simulink model "ID_3d_pend"  (R2023a)
settings: Solver=VariableStepAuto  StartTime=0.0  StopTime=1  RelTol=1e-9  AbsTol=1e-9  EnableMultiTasking=on
values from neighbouring files (symbols this model uses):
  a_el = [r_ej,h_ej,r_ej]    [data.m]
  akt = [0.5,0.5]*1    [inverse_dynamics.m]    (also in odvozeni_svaly.m = sym('akt',[1 3]))
  ax = r_ej    (= 0.088)    [data.m]
  ay = h_ej    (= 0.15)    [data.m]
  az = r_ej    (= 0.088)    [data.m]
  ccom = [-0.0110972, 0.00637508, 0.0541825]    [data.m]    (also in fo_python_to_matlab.m = [ccomx, ccomy, ccomz]; mm_python_to_matlab.m = [ccomx, ccomy, ccomz])
  cI = [5.75482e-05, 6.05521e-05, 1.05345e-05,-1.27405e-05, 1.65861e-05, 4.50136e-06]    [data.m]    (also in mm_python_to_matlab.m = [cixx, ciyy, cizz, cixy, ciyz, cizx])
  cont1 = [-0.083529 -0.01368 -0.098954]-scom    [data.m]
  cont2 = [-0.105456 -0.125076 -0.075251]-scom    [data.m]
  cont_params = [k_contact, eps]    [data.m]
  force = [556.8,1098.4]    [inverse_dynamics.m]    (also in odvozeni_svaly.m = (((length / l0m)^3) * exp(8 * length / l0m - 12.9) + (exp(-()
  h_ej = 0.15    [data.m]
  hcom = [0.000389382, -0.116338, -0.00231072]    [data.m]    (also in fo_python_to_matlab.m = [hcomx, hcomy, hcomz]; mm_python_to_matlab.m = [hcomx, hcomy, hcomz])
  hI = [0.00326632, 4.34807e-05, 0.00325004,-0.000136456, -1.30958e-06, -1.14964e-05]    [data.m]    (also in mm_python_to_matlab.m = [hixx, hiyy, hizz, hixy, hiyz, hizx])
  initialConditions = zeros(1,18)    [inverse_dynamics.m]
  k_contact = 10000    [data.m]
  l0m = [0.152404782147249,0.0902153118932702]    [inverse_dynamics.m]
  m = [0.0370005,0.12759,0.26363]    [data.m]    (also in fo_python_to_matlab.m = [c_m,s_m,h_m]; mm_python_to_matlab.m = [c_m,s_m,h_m])
  m_el = [x_ej,y_ej,z_ej]    [data.m]
  mx = x_ej    (= -0.03)    [data.m]
  my = y_ej    (= -0.1)    [data.m]
  mz = z_ej    (= 0.05)    [data.m]
  p = [c,k,g]    [data.m]    (also in fo_python_to_matlab.m)
  r_ej = 0.088    [data.m]
  scom = [-0.0512948, -0.0367122, -0.0430756]    [data.m]    (also in fo_python_to_matlab.m = [scomx, scomy, scomz]; mm_python_to_matlab.m = [scomx, scomy, scomz])
  sI = [0.00020065, 0.000202939, 0.000227237,-4.55661e-05, -7.53511e-05, -7.42694e-05]    [data.m]    (also in mm_python_to_matlab.m = [sixx, siyy, sizz, sixy, siyz, sizx])
  T_c = [-0.01433 0.02007 0.135535]    [data.m]    (also in fo_python_to_matlab.m = [T_cx,T_cy,T_cz]; mm_python_to_matlab.m = [T_cx,T_cy,T_cz]; odvozeni_svaly.m)
  T_d = 1e-20    [data.m]
  T_s = [-0.00955 -0.034 0.009]    [data.m]    (also in fo_python_to_matlab.m = [T_sx,T_sy,T_sz]; mm_python_to_matlab.m = [T_sx,T_sy,T_sz]; odvozeni_svaly.m)
  T_t = [0.006325 0.00693 0.025465]    [data.m]    (also in odvozeni_svaly.m)
  x_ej = -0.03    [data.m]
  y_ej = -0.1    [data.m]
  z_ej = 0.05    [data.m]
undefined symbols (not defined in the file or in its folder): phi_0, r_0, r_10, r_20, X, Y, Z
libraries: sm_lib x68, nesl_utility x43
(part 3 of 3)

== matlab function ID_3d_pend/MATLAB Function1 ==
  data: t input; q output
function q  = fcn(t)
% 
q = 0.2*cos(3*t)-0.1;
% dq = -0.5*sin(1*t);
% ddq = -0.5*cos(1*t);
% q = 0;
% dq = 0;
% ddq = 0;

== matlab function ID_3d_pend/scapulohumeral_rhythm/1_point_contact/r = fcn(h) ==
  data: h input; r output; h_ej parameter; r_ej parameter
function r = fcn(h,h_ej,r_ej)

r = sqrt((r_ej^2)*(1-h^2/h_ej^2));

== matlab function ID_3d_pend/scapulohumeral_rhythm/2_points_contact/ellipsoidal_joint_1/r = fcn(h) ==
  data: h input; r output; h_ej parameter; r_ej parameter
function r = fcn(h,h_ej,r_ej)

r = sqrt((r_ej^2)*(1-h^2/h_ej^2));

== matlab function ID_3d_pend/scapulohumeral_rhythm/2_points_contact/ellipsoidal_joint_2/r = fcn(h) ==
  data: h input; r output; h_ej parameter; r_ej parameter
function r = fcn(h,h_ej,r_ej)

r = sqrt((r_ej^2)*(1-h^2/h_ej^2));

== matlab function ID_3d_pend/MATLAB Function2 ==
  data: x1 input; xx output; x2 input; x3 input; x4 input; x5 input; x6 input; T_t parameter; T_c parameter; scom parameter; cont1 parameter; cont2 parameter; k_contact parameter; eps parameter; ax parameter; ay parameter; az parameter; mx parameter; my parameter; mz parameter
function xx = fcn(x1,x2,x3,x4,x5,x6,T_t, T_c, scom,cont1,cont2,k_contact, eps, ax, ay, az, mx, my, mz)
T_tx=T_t(1);
T_ty=T_t(2);
T_tz=T_t(3);
T_cx = T_c(1);
T_cy = T_c(2);
T_cz = T_c(3);
scomx = scom(1);
scomy = scom(2);
scomz = scom(3);
x_cont1 = cont1(1);
y_cont1 = cont1(2);
z_cont1 = cont1(3);
x_cont2 = cont2(1);
y_cont2 = cont2(2);
z_cont2 = cont2(3);

xx = -k_contact.*(ax.^2 + ay.^2 + az.^2).*(-0.5*sqrt(eps.^2 + (-1 + (T_cx.*(sin(x1).*sin(x3) - sin(x2).*cos(x1).*cos(x3)) + T_cy.*(sin(x1).*cos(x3) + sin(x2).*sin(x3).*cos(x1)) + T_cz.*cos(x1).*cos(x2) + T_tz - mz + scomx.*((sin(x1).*sin(x3) - sin(x2).*cos(x1).*cos(x3)).*cos(x5).*cos(x6) + (sin(x1).*cos(x3) + sin(x2).*sin(x3).*cos(x1)).*(sin(x4).*sin(x5).*cos(x6) + sin(x6).*cos(x4)) + (sin(x4).*sin(x6) - sin(x5).*cos(x4).*cos(x6)).*cos(x1).*cos(x2)) + scomy.*(-(sin(x1).*sin(x3) - sin(x2).*cos(x1).*cos(x3)).*sin(x6).*cos(x5) + (sin(x1).*cos(x3) + sin(x2).*sin(x3).*cos(x1)).*(-sin(x4).*sin(x5).*sin(x6) + cos(x4).*cos(x6)) + (sin(x4).*cos(x6) + sin(x5).*sin(x6).*cos(x4)).*cos(x1).*cos(x2)) + scomz.*((sin(x1).*sin(x3) - sin(x2).*cos(x1).*cos(x3)).*sin(x5) - (sin(x1).*cos(x3) + sin(x2).*sin(x3).*cos(x1)).*sin(x4).*cos(x5) + cos(x1).*cos(x2).*cos(x4).*cos(x5)) + x_cont1.*((sin(x1).*sin(x3) - sin(x2).*cos(x1).*cos(x3)).*cos(x5).*cos(x6) + (sin(x1).*cos(x3) + sin(x2).*sin(x3).*cos(x1)).*(sin(x4).*sin(x5).*cos(x6) + sin(x6).*cos(x4)) + (sin(x4).*sin(x6) - sin(x5).*cos(x4).*cos(x6)).*cos(x1).*cos(x2)) + y_cont1.*(-(sin(x1).*sin(x3) - sin(x2).*cos(x1).*cos(x3)).*sin(x6).*cos(x5) + (sin(x1).*cos(x3) + sin(x2).*sin(x3).*cos(x1)).*(-sin(x4).*sin(x5).*sin(x6) + cos(x4).*cos(x6)) + (sin(x4).*cos(x6) + sin(x5).*sin(x6).*cos(x4)).*cos(x1).*cos(x2)) + z_cont1.*((sin(x1).*sin(x3) - sin(x2).*cos(x1).*cos(x3)).*sin(x5) - (sin(x1).*cos(x3) + sin(x2).*sin(x3).*cos(x1)).*sin(x4).*cos(x5) + cos(x1).*cos(x2).*cos(x4).*cos(x5))).^2./az.^2 + (T_cx.*(sin(x1).*sin(x2).*cos(x3) + sin(x3).*cos(x1)) + T_cy.*(-sin(x1).*sin(x2).*sin(x3) + cos(x1).*cos(x3)) - T_cz.*sin(x1).*cos(x2) + T_ty - my + scomx.*(-(sin(x4).*sin(x6) - sin(x5).*cos(x4).*cos(x6)).*sin(x1).*cos(x2) + (-sin(x1).*sin(x2).*sin(x3) + cos(x1).*cos(x3)).*(sin(x4).*sin(x5).*cos(x6) + sin(x6).*cos(x4)) + (sin(x1).*sin(x2).*cos(x3) + sin(x3).*cos(x1)).*cos(x5).*cos(x6)) + scomy.*(-(sin(x4).*cos(x6) + sin(x5).*sin(x6).*cos(x4)).*sin(x1).*cos(x2) + (-sin(x1).*sin(x2).*sin(x3) + cos(x1).*cos(x3)).*(-sin(x4).*sin(x5).*sin(x6) + cos(x4).*cos(x6)) - (sin(x1).*sin(x2).*cos(x3) + sin(x3).*cos(x1)).*sin(x6).*cos(x5)) + scomz.*(-(-sin(x1).*sin(x2).*sin(x3) + cos(x1).*cos(x3)).*sin(x4).*cos(x5) + (sin(x1).*sin(x2).*cos(x3) + sin(x3).*cos(x1)).*sin(x5) - sin(x1).*cos(x2).*cos(x4).*cos(x5)) + x_cont1.*(-(sin(x4).*sin(x6) - sin(x5).*cos(x4).*cos(x6)).*sin(x1).*cos(x2) + (-sin(x1).*sin(x2).*sin(x3) + cos(x1).*cos(x3)).*(sin(x4).*sin(x5).*cos(x6) + sin(x6).*cos(x4)) + (sin(x1).*sin(x2).*cos(x3) + sin(x3).*cos(x1)).*cos(x5).*cos(x6)) + y_cont1.*(-(sin(x4).*cos(x6) + sin(x5).*sin(x6).*cos(x4)).*sin(x1).*cos(x2) + (-sin(x1).*sin(x2).*sin(x3) + cos(x1).*cos(x3)).*(-sin(x4).*sin(x5).*sin(x6) + cos(x4).*cos(x6)) - (sin(x1).*sin(x2).*cos(x3) + sin(x3).*cos(x1)).*sin(x6).*cos(x5)) + z_cont1.*(-(-sin(x1).*sin(x2).*sin(x3) + cos(x1).*cos(x3)).*sin(x4).*cos(x5) + (sin(x1).*sin(x2).*cos(x3) + sin(x3).*cos(x1)).*sin(x5) - sin(x1).*cos(x2).*cos(x4).*cos(x5))).^2./ay.^2 + (T_cx.*cos(x2).*cos(x3) - T_cy.*sin(x3).*cos(x2) + T_cz.*sin(x2) + T_tx - mx + scomx.*((sin(x4).*sin(x6) - sin(x5).*cos(x4).*cos(x6)).*sin(x2) - (sin(x4).*sin(x5).*cos(x6) + sin(x6).*cos(x4)).*sin(x3).*cos(x2) + cos(x2).*cos(x3).*cos(x5).*cos(x6)) + scomy.*((sin(x4).*cos(x6) + sin(x5).*sin(x6).*cos(x4)).*sin(x2) - (-sin(x4).*sin(x5).*sin(x6) + cos(x4).*cos(x6)).*sin(x3).*cos(x2) - sin(x6).*cos(x2).*cos(x3).*cos(x5)) + scomz.*(sin(x2).*cos(x4).*cos(x5) + sin(x3).*sin(x4).*cos(x2).*cos(x5) + sin(x5).*cos(x2).*cos(x3)) + x_cont1.*((sin(x4).*sin(x6) - sin(x5).*cos(x4).*cos(x6)).*sin(x2) - (sin(x4).*sin(x5).*cos(x6) + sin(x6).*cos(x4)).*sin(x3).*cos(x2) + cos(x2).*cos(x3).*cos(x5).*cos(x6)) + y_cont1.*((sin(x4).*cos(x6) + sin(x5).*sin(x6).*cos(x4)).*sin(x2) - (-sin(x4).*sin(x5).*sin(x6) + cos(x4).*cos(x6)).*sin(x3).*cos(x2) - sin(x6).*cos(x2).*cos(x3).*cos(x5)) + z_cont1.*(sin(x2).*cos(x4).*cos(x5) + sin(x3).*sin(x4).*cos(x2).*cos(x5) + sin(x5).*cos(x2).*cos(x3))).^2./ax.^2).^2) - 0.5 + 0.5*(T_cx.*(sin(x1).*sin(x3) - sin(x2).*cos(x1).*cos(x3)) + T_cy.*(sin(x1).*cos(x3) + sin(x2).*sin(x3).*cos(x1)) + T_cz.*cos(x1).*cos(x2) + T_tz - mz + scomx.*((sin(x1).*sin(x3) - sin(x2).*cos(x1).*cos(x3)).*cos(x5).*cos(x6) + (sin(x1).*cos(x3) + sin(x2).*sin(x3).*cos(x1)).*(sin(x4).*sin(x5).*cos(x6) + sin(x6).*cos(x4)) + (sin(x4).*sin(x6) - sin(x5).*cos(x4).*cos(x6)).*cos(x1).*cos(x2)) + scomy.*(-(sin(x1).*sin(x3) - sin(x2).*cos(x1).*cos(x3)).*sin(x6).*cos(x5) + (sin(x1).*cos(x3) + sin(x2).*sin(x3).*cos(x1)).*(-sin(x4).*sin(x5).*sin(x6) + cos(x4).*cos(x6)) + (sin(x4).*cos(x6) + sin(x5).*sin(x6).*cos(x4)).*cos(x1).*cos(x2)) + scomz.*((sin(x1).*sin(x3) - sin(x2).*cos(x1).*cos(x3)).*sin(x5) - (sin(x1).*cos(x3) + sin(x2).*sin(x3).*cos(x1)).*sin(x4).*cos(x5) + cos(x1).*cos(x2).*cos(x4).*cos(x5)) + x_cont1.*((sin(x1).*sin(x3) - sin(x2).*cos(x1).*cos(x3)).*cos(x5).*cos(x6) + (sin(x1).*cos(x3) + sin(x2).*sin(x3).*cos(x1)).*(sin(x4).*sin(x5).*cos(x6) + sin(x6).*cos(x4)) + (sin(x4).*sin(x6) - sin(x5).*cos(x4).*cos(x6)).*cos(x1).*cos(x2)) + y_cont1.*(-(sin(x1).*sin(x3) - sin(x2).*cos(x1).*cos(x3)).*sin(x6).*cos(x5) + (sin(x1).*cos(x3) + sin(x2).*sin(x3).*cos(x1)).*(-sin(x4).*sin(x5).*sin(x6) + cos(x4).*cos(x6)) + (sin(x4).*cos(x6) + sin(x5).*sin(x6).*cos(x4)).*cos(x1).*cos(x2)) + z_cont1.*((sin(x1).*sin(x3) - sin(x2).*cos(x1).*cos(x3)).*sin(x5) - (sin(x1).*cos(x3) + sin(x2).*sin(x3).*cos(x1)).*sin(x4).*cos(x5) + cos(x1).*cos(x2).*cos(x4).*cos(x5))).^2./az.^2 + 0.5*(T_cx.*(sin(x1).*sin(x2).*cos(x3) + sin(x3).*cos(x1)) + T_cy.*(-sin(x1).*sin(x2).*sin(x3) + cos(x1).*cos(x3)) - T_cz.*sin(x1).*cos(x2) + T_ty - my + scomx.*(-(sin(x4).*sin(x6) - sin(x5).*cos(x4).*cos(x6)).*sin(x1).*cos(x2) + (-sin(x1).*sin(x2).*sin(x3) + cos(x1).*cos(x3)).*(sin(x4).*sin(x5).*cos(x6) + sin(x6).*cos(x4)) + (sin(x1).*sin(x2).*cos(x3) + sin(x3).*cos(x1)).*cos(x5).*cos(x6)) + scomy.*(-(sin(x4).*cos(x6) + sin(x5).*sin(x6).*cos(x4)).*sin(x1).*cos(x2) + (-sin(x1).*sin(x2).*sin(x3) + cos(x1).*cos(x3)).*(-sin(x4).*sin(x5).*sin(x6) + cos(x4).*cos(x6)) - (sin(x1).*sin(x2).*cos(x3) + sin(x3).*cos(x1)).*sin(x6).*cos(x5)) + scomz.*(-(-sin(x1).*sin(x2).*sin(x3) + cos(x1).*cos(x3)).*sin(x4).*cos(x5) + (sin(x1).*sin(x2).*cos(x3) + sin(x3).*cos(x1)).*sin(x5) - sin(x1).*cos(x2).*cos(x4).*cos(x5)) + x_cont1.*(-(sin(x4).*sin(x6) - sin(x5).*cos(x4).*cos(x6)).*sin(x1).*cos(x2) + (-sin(x1).*sin(x2).*sin(x3) + cos(x1).*cos(x3)).*(sin(x4).*sin(x5).*cos(x6) + sin(x6).*cos(x4)) + (sin(x1).*sin(x2).*cos(x3) + sin(x3).*cos(x1)).*cos(x5).*cos(x6)) + y_cont1.*(-(sin(x4).*cos(x6) + sin(x5).*sin(x6).*cos(x4)).*sin(x1).*cos(x2) + (-sin(x1).*sin(x2).*sin(x3) + cos(x1).*cos(x3)).*(-sin(x4).*sin(x5).*sin(x6) + cos(x4).*cos(x6)) - (sin(x1).*sin(x2).*cos(x3) + sin(x3).*cos(x1)).*sin(x6).*cos(x5)) + z_cont1.*(-(-sin(x1).*sin(x2).*sin(x3) + cos(x1).*cos(x3)).*sin(x4).*cos(x5) + (sin(x1).*sin(x2).*cos(x3) + sin(x3).*cos(x1)).*sin(x5) - sin(x1).*cos(x2).*cos(x4).*cos(x5))).^2./ay.^2 + 0.5*(T_cx.*cos(x2).*cos(x3) - T_cy.*sin(x3).*cos(x2) + T_cz.*sin(x2) + T_tx - mx + scomx.*((sin(x4).*sin(x6) - sin(x5).*cos(x4).*cos(x6)).*sin(x2) - (sin(x4).*sin(x5).*cos(x6) + sin(x6).*cos(x4)).*sin(x3).*cos(x2) + cos(x2).*cos(x3).*cos(x5).*cos(x6)) + scomy.*((sin(x4).*cos(x6) + sin(x5).*sin(x6).*cos(x4)).*sin(x2) - (-sin(x4).*sin(x5).*sin(x6) + cos(x4).*cos(x6)).*sin(x3).*cos(x2) - sin(x6).*cos(x2).*cos(x3).*cos(x5)) + scomz.*(sin(x2).*cos(x4).*cos(x5) + sin(x3).*sin(x4).*cos(x2).*cos(x5) + sin(x5).*cos(x2).*cos(x3)) + x_cont1.*((sin(x4).*sin(x6) - sin(x5).*cos(x4).*cos(x6)).*sin(x2) - (sin(x4).*sin(x5).*cos(x6) + sin(x6).*cos(x4)).*sin(x3).*cos(x2) + cos(x2).*cos(x3).*cos(x5).*cos(x6)) + y_cont1.*((sin(x4).*cos(x6) + sin(x5).*sin(x6).*cos(x4)).*sin(x2) - (-sin(x4).*sin(x5).*sin(x6) + cos(x4).*cos(x6)).*sin(x3).*cos(x2) - sin(x6).*cos(x2).*cos(x3).*cos(x5)) + z_cont1.*(sin(x2).*cos(x4).*cos(x5) + sin(x3).*sin(x4).*cos(x2).*cos(x5) + sin(x5).*cos(x2).*cos(x3))).^2./ax.^2).*(T_cx.*(sin(x1).*sin(x3) - sin(x2).*cos(x1).*cos(x3)) + T_cy.*(sin(x1).*cos(x3) + sin(x2).*sin(x3).*cos(x1)) + T_cz.*cos(x1).*cos(x2) + T_tz - mz + scomx.*((sin(x1).*sin(x3) - sin(x2).*cos(x1).*cos(x3)).*cos(x5).*cos(x6) + (sin(x1).*cos(x3) + sin(x2).*sin(x3).*cos(x1)).*(sin(x4).*sin(x5).*cos(x6) + sin(x6).*cos(x4)) + (sin(x4).*sin(x6) - sin(x5).*cos(x4).*cos(x6)).*cos(x1).*cos(x2)) + scomy.*(-(sin(x1).*sin(x3) - sin(x2).*cos(x1).*cos(x3)).*sin(x6).*cos(x5) + (sin(x1).*cos(x3) + sin(x2).*sin(x3).*cos(x1)).*(-sin(x4).*sin(x5).*sin(x6) + cos(x4).*cos(x6)) + (sin(x4).*cos(x6) + sin(x5).*sin(x6).*cos(x4)).*cos(x1).*cos(x2)) + scomz.*((sin(x1).*sin(x3) - sin(x2).*cos(x1).*cos(x3)).*sin(x5) - (sin(x1).*cos(x3) + sin(x2).*sin(x3).*cos(x1)).*sin(x4).*cos(x5) + cos(x1).*cos(x2).*cos(x4).*cos(x5)) + x_cont1.*((sin(x1).*sin(x3) - sin(x2).*cos(x1).*cos(x3)).*cos(x5).*cos(x6) + (sin(x1).*cos(x3) + sin(x2).*sin(x3).*cos(x1)).*(sin(x4).*sin(x5).*cos(x6) + sin(x6).*cos(x4)) + (sin(x4).*sin(x6) - sin(x5).*cos(x4).*cos(x6)).*cos(x1).*cos(x2)) + y_cont1.*(-(sin(x1).*sin(x3) - sin(x2).*cos(x1).*cos(x3)).*sin(x6).*cos(x5) + (sin(x1).*cos(x3) + sin(x2).*sin(x3).*cos(x1)).*(-sin(x4).*sin(x5).*sin(x6) + cos(x4).*cos(x6)) + (sin(x4).*cos(x6) + sin(x5).*sin(x6).*cos(x4)).*cos(x1).*cos(x2)) + z_cont1.*((sin(x1).*sin(x3) - sin(x2).*cos(x1).*cos(x3)).*sin(x5) - (sin(x1).*cos(x3) + sin(x2).*sin(x3).*cos(x1)).*sin(x4).*cos(x5) + cos(x1).*cos(x2).*cos(x4).*cos(x5)))./az.^2;

== matlab function ID_3d_pend/scapulohumeral_rhythm/Subsystem/point 1/F ==
  data: x input; Fx output; y input; z input; Fy output; Fz output; x_ej parameter; y_ej parameter; z_ej parameter; r_ej parameter; h_ej parameter; eps parameter; k_contact parameter
function [Fx,Fy,Fz]= fcn(x,y,z,x_ej, y_ej, z_ej, r_ej, h_ej, eps, k_contact)

f = ((x-x_ej)/r_ej)^2+((y-y_ej)/h_ej)^2+((z-z_ej)/r_ej)^2-1;
F = 1/2*(f-sqrt(f^2+eps^2));

Fx = -k_contact*(x-x_ej)*(r_ej^2+h_ej^2+r_ej^2)/(r_ej^2)*F;
Fy = -k_contact*(y-y_ej)*(r_ej^2+h_ej^2+r_ej^2)/(h_ej^2)*F;
Fz = -k_contact*(z-z_ej)*(r_ej^2+h_ej^2+r_ej^2)/(r_ej^2)*F;

%% 2D
% 
% f = ((x-mx)/ax)^2+((z-mz)/az)^2-1;
% F = 1/2*(f-sqrt(f^2+eps^2));
% 
% Fx = -k*(x-mx)*(ax^2+ay^2)/(ax^2)*F;
% Fy = -k*(y-my)*(ax^2+ay^2)/(ay^2)*F;
% Fz = -k*(z-mz)*(ax^2+ay^2)/(az^2)*F;

== matlab function ID_3d_pend/scapulohumeral_rhythm/Subsystem/point 2/F ==
  data: x input; Fx output; y input; z input; Fy output; Fz output; x_ej parameter; y_ej parameter; z_ej parameter; r_ej parameter; h_ej parameter; eps parameter; k_contact parameter
function [Fx,Fy,Fz]= fcn(x,y,z,x_ej, y_ej, z_ej, r_ej, h_ej, eps, k_contact)

f = ((x-x_ej)/r_ej)^2+((y-y_ej)/h_ej)^2+((z-z_ej)/r_ej)^2-1;
F = 1/2*(f-sqrt(f^2+eps^2));

Fx = -k_contact*(x-x_ej)*(r_ej^2+h_ej^2+r_ej^2)/(r_ej^2)*F;
Fy = -k_contact*(y-y_ej)*(r_ej^2+h_ej^2+r_ej^2)/(h_ej^2)*F;
Fz = -k_contact*(z-z_ej)*(r_ej^2+h_ej^2+r_ej^2)/(r_ej^2)*F;

%% 2D
% 
% f = ((x-mx)/ax)^2+((z-mz)/az)^2-1;
% F = 1/2*(f-sqrt(f^2+eps^2));
% 
% Fx = -k*(x-mx)*(ax^2+ay^2)/(ax^2)*F;
% Fy = -k*(y-my)*(ax^2+ay^2)/(ay^2)*F;
% Fz = -k*(z-mz)*(ax^2+ay^2)/(az^2)*F;

== matlab function ID_3d_pend/DELT1/Active_factor_norm ==
  data: Fa_norm output; lm input; l0 input; a input
function Fa_norm = fcn(lm,l0,a)
f_gauss = 0.25;
Fa_norm = (exp(-(lm/l0-1)^2/f_gauss))*a;

== matlab function ID_3d_pend/scapulohumeral_rhythm/1_point_contact/phi = fcn(h) ==
  data: h input; phi output; h_ej parameter; r_ej parameter
function phi = fcn(h,h_ej,r_ej)

phi = atan(-(r_ej*h)/(h_ej^2*sqrt(1-h^2/h_ej^2)));

== matlab function ID_3d_pend/DELT1/Passive_force_norm ==
  data: lm input; Fp_norm output; l0 input
function Fp_norm = fcn(lm,l0)
Fp_norm = ((lm/l0)^3)*exp(8*lm/l0-12.9);

== matlab function ID_3d_pend/DELT2/Active_factor_norm ==
  data: Fa_norm output; lm input; l0 input; a input
function Fa_norm = fcn(lm,l0,a)
f_gauss = 0.25;
Fa_norm = (exp(-(lm/l0-1)^2/f_gauss))*a;

== matlab function ID_3d_pend/DELT2/Passive_force_norm ==
  data: lm input; Fp_norm output; l0 input
function Fp_norm = fcn(lm,l0)
Fp_norm = ((lm/l0)^3)*exp(8*lm/l0-12.9);

== matlab function ID_3d_pend/Pect2/Active_factor_norm ==
  data: Fa_norm output; lm input; l0 input; a input
function Fa_norm = fcn(lm,l0,a)
f_gauss = 0.25;
Fa_norm = (exp(-(lm/l0-1)^2/f_gauss))*a;

== matlab function ID_3d_pend/Pect2/Passive_force_norm ==
  data: lm input; Fp_norm output; l0 input
function Fp_norm = fcn(lm,l0)
Fp_norm = ((lm/l0)^3)*exp(8*lm/l0-12.9);

== matlab function ID_3d_pend/MATLAB Function ==
  data: t input; q input; dq input; ddq input; m parameter; y output; cI parameter; sI parameter; hI parameter; ccom parameter; scom parameter; hcom parameter; T_c parameter; T_s parameter; p parameter; akt parameter; T_t parameter; m_el parameter; a_el parameter; cont1 parameter; cont2 parameter; cont_params parameter
function y = fcn(t,q,dq,ddq,m,cI,sI,hI,ccom,scom,hcom,T_c,T_s,p,akt,T_t, m_el, a_el, cont1, cont2, cont_params)
y = zeros(18,1);
y = fcn_ID(t,q,dq,ddq,m,cI,sI,hI,ccom,scom,hcom,T_t,T_c,T_s,p,m_el,a_el,cont1,cont2,cont_params,akt);
